simulink model "halfsubtractor"  (R2025b)
settings: Solver=VariableStepAuto  StartTime=0.0  StopTime=10.0  RelTol=1e-3
settings Model: Creator=cyber  LastModifiedBy=cyber

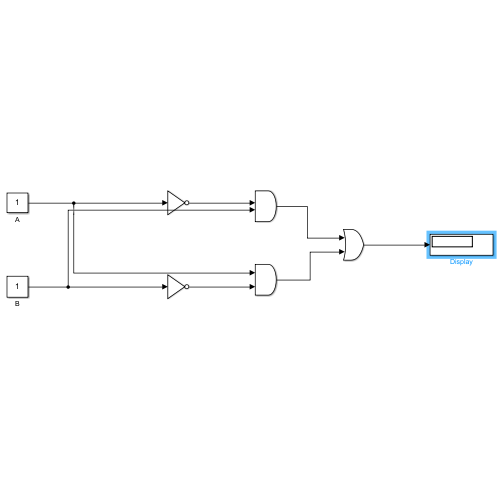
[thumbnail: Simulink's stored preview of the top-level diagram]
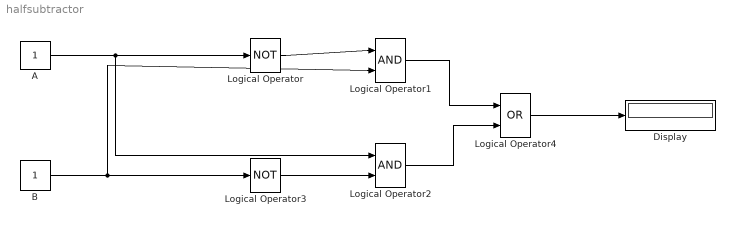
== system halfsubtractor ==
  A : Constant
  B : Constant
  Display : Display
  Logical Operator : Logic  Operator=NOT  IconShape=distinctive  AllPortsSameDT=off  OutDataTypeStr=boolean
  Logical Operator1 : Logic  IconShape=distinctive  AllPortsSameDT=off  OutDataTypeStr=boolean
  Logical Operator2 : Logic  IconShape=distinctive  AllPortsSameDT=off  OutDataTypeStr=boolean
  Logical Operator3 : Logic  Operator=NOT  IconShape=distinctive  AllPortsSameDT=off  OutDataTypeStr=boolean
  Logical Operator4 : Logic  Operator=OR  IconShape=distinctive  AllPortsSameDT=off  OutDataTypeStr=boolean
  wires:
  A/1 -> Logical Operator2/1, Logical Operator/1
  Logical Operator/1 -> Logical Operator1/1
  B/1 -> Logical Operator1/2, Logical Operator3/1
  Logical Operator3/1 -> Logical Operator2/2
  Logical Operator1/1 -> Logical Operator4/1
  Logical Operator2/1 -> Logical Operator4/2
  Logical Operator4/1 -> Display/1
